simulink model "main"  (R2017b)
settings: Solver=VariableStepAuto  StartTime=0.0  StopTime=0.25  FixedStep=2e-4  RelTol=1e-3
values from neighbouring files (symbols this model uses):
  accCoef = 0    [initiateSimulation.m]
  idealAccCoef = sum(m)    [initiateSimulation.m]
  idealJerkCoef = sum(m) * tau    [initiateSimulation.m]
  idealSnapCoef = sum(m) * ( 1/wn.^2 + 0.5 * tau.^2)    [initiateSimulation.m]
  jerkCoef = 0    [initiateSimulation.m]
  kd = tempPD.Kd    [Untitled3.m]
  ki = tempPD.Ki    [Untitled3.m]
  kp = tempPD.Kp    [Untitled3.m]
  snapCoef = 0    [initiateSimulation.m]
  tau = 1.5*Ts    (= 0.0003)    [initiateSimulation.m]
  Ts = 1/fs    (= 0.0002)    [initiateSimulation.m]
undefined symbols (not defined in the file or in its folder): kdScale
libraries: model_controller x3, simulink x2, cstblocks x2
settings Model: Creator=Dai Luyao  LastModifiedBy=Princess
settings CodeAppCC: StateflowObjectComments=on

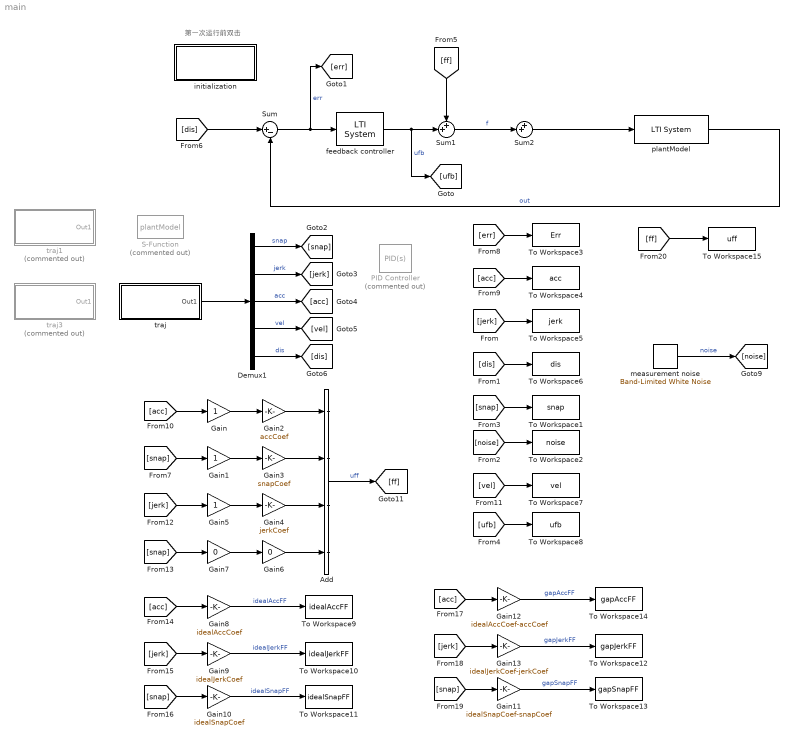
== system main ==
  note: 第一次运行前双击
  Add : Sum  Inputs=++++
  Demux1 : Demux  Outputs=5
  Gain : Gain
  Gain1 : Gain
  Gain10 : Gain  Gain=idealSnapCoef
  Gain11 : Gain  Gain=idealSnapCoef-snapCoef
  Gain12 : Gain  Gain=idealAccCoef-accCoef
  Gain13 : Gain  Gain=idealJerkCoef-jerkCoef
  Gain2 : Gain  Gain=accCoef
  Gain3 : Gain  Gain=snapCoef
  Gain4 : Gain  Gain=jerkCoef
  Gain5 : Gain
  Gain6 : Gain  Gain=0
  Gain7 : Gain  Gain=0
  Gain8 : Gain  Gain=idealAccCoef
  Gain9 : Gain  Gain=idealJerkCoef
  PID Controller : simulink/Continuous/PID Controller  Commented=on  Controller=PID  TimeDomain=Continuous-time  SampleTime=-1  IntegratorMethod=Forward Euler  FilterMethod=Forward Euler  Form=Parallel  UseFilter=on  ControllerParametersSource=internal  P=kp  I=1.5*ki  D=kdScale * kd  N=1/tau  InitialConditionSource=internal  InitialConditionForIntegrator=0  InitialConditionForFilter=0  ExternalReset=none  LimitOutput=off  UpperSaturationLimit=inf  LowerSaturationLimit=-inf  LinearizeAsGain=on  AntiWindupMode=none  Kb=1  TrackingMode=off  Kt=1  PParamMin=[]  PParamMax=[]  IParamMin=[]  IParamMax=[]  DParamMin=[]  DParamMax=[]  NParamMin=[]  NParamMax=[]  KbParamMin=[]  KbParamMax=[]  KtParamMin=[]  KtParamMax=[]  POutMin=[]  POutMax=[]  IOutMin=[]  IOutMax=[]  DOutMin=[]  DOutMax=[]  NOutMin=[]  NOutMax=[]  KbOutMin=[]  KbOutMax=[]  KtOutMin=[]  KtOutMax=[]  IntegratorOutMin=[]  IntegratorOutMax=[]  FilterOutMin=[]  FilterOutMax=[]  SumOutMin=[]  SumOutMax=[]  SumI1OutMin=[]  SumI1OutMax=[]  SumI2OutMin=[]  SumI2OutMax=[]  SumI3OutMin=[]  SumI3OutMax=[]  SumDOutMin=[]  SumDOutMax=[]  SaturationOutMin=[]  SaturationOutMax=[]  IntegratorContinuousStateAttributes=''  IntegratorStateMustResolveToSignalObject=off  IntegratorRTWStateStorageClass=Auto  FilterContinuousStateAttributes=''  FilterStateMustResolveToSignalObject=off  FilterRTWStateStorageClass=Auto  DifferentiatorICPrevScaledInput=0  DifferentiatorOutMin=[]  DifferentiatorOutMax=[]  InitialConditionSetting=State (most efficient)  FilterDiffOutCoefMin=[]  FilterDiffOutCoefMax=[]  SumDenOutMin=[]  SumDenOutMax=[]  SumNumOutMin=[]  SumNumOutMax=[]  ReciprocalOutMin=[]  ReciprocalOutMax=[]  DivideOutMin=[]  DivideOutMax=[]  TunerSelectOption=Transfer Function Based (PID Tuner App)
  S-Function : S-Function  Commented=on  FunctionName=plantModel  Parameters=modelParameters  SFunctionDeploymentMode=off  EnableBusSupport=off
  Sum : Sum  Inputs=|+-
  Sum1 : Sum  Inputs=++|
  Sum2 : Sum  Inputs=++|
  To Workspace1 : ToWorkspace  VariableName=snap  SaveFormat=Structure With Time  SampleTime=Ts
  To Workspace10 : ToWorkspace  VariableName=idealJerkFF  SaveFormat=Timeseries  SampleTime=Ts
  To Workspace11 : ToWorkspace  VariableName=idealSnapFF  SaveFormat=Timeseries  SampleTime=Ts
  To Workspace12 : ToWorkspace  VariableName=gapJerkFF  SaveFormat=Timeseries  SampleTime=Ts
  To Workspace13 : ToWorkspace  VariableName=gapSnapFF  SaveFormat=Timeseries  SampleTime=Ts
  To Workspace14 : ToWorkspace  VariableName=gapAccFF  SaveFormat=Timeseries  SampleTime=Ts
  To Workspace15 : ToWorkspace  VariableName=uff  SaveFormat=Structure With Time  SampleTime=Ts
  To Workspace2 : ToWorkspace  VariableName=noise  SaveFormat=Structure With Time  SampleTime=Ts
  To Workspace3 : ToWorkspace  VariableName=Err  SaveFormat=Structure With Time  SampleTime=Ts
  To Workspace4 : ToWorkspace  VariableName=acc  SaveFormat=Structure With Time  SampleTime=Ts
  To Workspace5 : ToWorkspace  VariableName=jerk  SaveFormat=Structure With Time  SampleTime=Ts
  To Workspace6 : ToWorkspace  VariableName=dis  SaveFormat=Structure With Time  SampleTime=Ts
  To Workspace7 : ToWorkspace  VariableName=vel  SaveFormat=Structure With Time  SampleTime=Ts
  To Workspace8 : ToWorkspace  VariableName=ufb  SaveFormat=Structure With Time  SampleTime=Ts
  To Workspace9 : ToWorkspace  VariableName=idealAccFF  SaveFormat=Timeseries  SampleTime=Ts
  feedback controller : cstblocks/LTI System  sys=Gc  IC=[]
  initialization : Subsystem
      settings: OpenFcn=initiateSimulation;  MoveFcn=edit initiateSimulation;
  measurement noise : simulink/Sources/Band-Limited White Noise  Cov=0  Ts=1e-5  seed=[23331]
  plantModel : cstblocks/LTI System  sys=Gp  IC=[]
  traj : Subsystem  BlockChoice=4th order traj
      link override 2nd order traj: x=0.6  v=0.25  a=10
      link override 3rd order traj: j=trajParameters.jerk  v=trajParameters.vel  x=trajParameters.dis  a=trajParameters.acc
      link override 4th order traj: a=trajParameters.acc  v=trajParameters.vel  x=trajParameters.dis  j=trajParameters.jerk  d=trajParameters.snap  Ts=0
      settings: AttributesFormatString=%<BlockChoice>  TemplateBlock=model_controller/Profile Generators/traj  MemberBlocks=2th order traj,3rd order traj,4th order traj,step
  traj1 : Subsystem  Commented=on  BlockChoice=4th order traj
      link override 2nd order traj: x=0.6  v=0.25  a=10
      link override 3rd order traj: j=2000  v=0.25  x=0.04  a=10
      link override 4th order traj: a=20  v=0.5  x=0.04  j=2000  d=1.5e6
      settings: AttributesFormatString=%<BlockChoice>  TemplateBlock=model_controller/Profile Generators/traj  MemberBlocks=2th order traj,3rd order traj,4th order traj,step
  traj3 : Subsystem  Commented=on  BlockChoice=4th order traj
      link override 2nd order traj: x=0.6  v=0.25  a=10
      link override 3rd order traj: j=2000  v=0.25  x=0.04  a=10
      link override 4th order traj: a=10  v=0.25  x=0.04  j=800  d=64000
      settings: AttributesFormatString=%<BlockChoice>  TemplateBlock=model_controller/Profile Generators/traj  MemberBlocks=2th order traj,3rd order traj,4th order traj,step
  wires:
  Sum/1 -> feedback controller/1, [err]  "err"
  measurement noise/1 -> [noise]  "noise"
  Demux1/1 -> [snap]  "snap"
  Demux1/2 -> [jerk]  "jerk"
  Demux1/3 -> [acc]  "acc"
  Demux1/4 -> [vel]  "vel"
  Demux1/5 -> [dis]  "dis"
  [acc] -> To Workspace4/1
  [acc] -> Gain/1
  [jerk] -> To Workspace5/1
  [dis] -> To Workspace6/1
  [err] -> To Workspace3/1
  [noise] -> To Workspace2/1
  [dis] -> Sum/1
  [ff] -> Sum1/1
  [snap] -> To Workspace1/1
  [snap] -> Gain1/1
  Gain/1 -> Gain2/1
  Gain1/1 -> Gain3/1
  Add/1 -> [ff]  "uff"
  Gain2/1 -> Add/1
  Gain3/1 -> Add/2
  [vel] -> To Workspace7/1
  Gain4/1 -> Add/3
  [jerk] -> Gain5/1
  Gain5/1 -> Gain4/1
  Gain7/1 -> Gain6/1
  [snap] -> Gain7/1
  Gain6/1 -> Add/4
  plantModel/1 -> Sum/2  "out"
  traj/1(Out1) -> Demux1/1
  feedback controller/1 -> [ufb], Sum1/2  "ufb"
  Sum1/1 -> Sum2/2  "f"
  Sum2/1 -> plantModel/1
  [ufb] -> To Workspace8/1
  [acc] -> Gain8/1
  [jerk] -> Gain9/1
  [snap] -> Gain10/1
  Gain8/1 -> To Workspace9/1  "idealAccFF"
  Gain10/1 -> To Workspace11/1  "idealSnapFF"
  Gain9/1 -> To Workspace10/1  "idealJerkFF"
  Gain13/1 -> To Workspace12/1  "gapJerkFF"
  Gain11/1 -> To Workspace13/1  "gapSnapFF"
  Gain12/1 -> To Workspace14/1  "gapAccFF"
  [snap] -> Gain11/1
  [jerk] -> Gain13/1
  [acc] -> Gain12/1
  [ff] -> To Workspace15/1

== system main/initialization ==

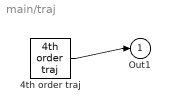
== system main/traj ==
  4th order traj : model_controller/Profile Generators/4th order traj  t0=0  x=trajParameters.dis  v=trajParameters.vel  a=trajParameters.acc  j=trajParameters.jerk  d=trajParameters.snap  Ts=0
  Out1 : Outport
  wires:
  4th order traj/1 -> Out1/1

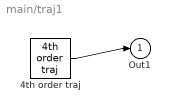
== system main/traj1 ==
  4th order traj : model_controller/Profile Generators/4th order traj  t0=0  x=0.04  v=0.5  a=20  j=2000  d=1.5e6  Ts=0
  Out1 : Outport
  wires:
  4th order traj/1 -> Out1/1

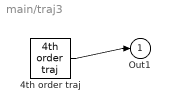
== system main/traj3 ==
  4th order traj : model_controller/Profile Generators/4th order traj  t0=0  x=0.04  v=0.25  a=10  j=800  d=64000  Ts=0
  Out1 : Outport
  wires:
  4th order traj/1 -> Out1/1
